simulink model "robobee_smoothSynchAsynch"  (R2021a)
settings: Solver=ode5  StartTime=0.0  StopTime=10  FixedStep=samptime  RelTol=1e-3
values from neighbouring files (symbols this model uses):
  Amplitude = 4    [robobee_simulink_script.m]
  den = [1 a2 a3]    [robobee_simulink_script.m]
  Frequency = 66    [robobee_simulink_script.m]
  num = [a1 0]    [robobee_simulink_script.m]
  pf = [0.0008   -0.0042    0.0029]    [robobee_simulink_script.m]
  samptime = 1/10000    (= 0.0001)    [robobee_simulink_script.m]
  t_end = 6+4    (= 10)    [robobee_simulink_script.m]
  t_switch = t_end/2    (= 5)    [robobee_simulink_script.m]
  VBias = 200/daq_to_piezo_volt    (= 8)    [robobee_simulink_script.m]
undefined symbols (not defined in the file or in its folder): National_Instruments, PCIe
libraries: sldrtlib x3, simulink x2, cstblocks x1
settings Model: SimulationMode=external  ExtModeTrigDuration=500000  Creator=Gravish Lab  LastModifiedBy=RoBeePC
settings SolverCC: AlgebraicLoopSolver=TrustRegion
settings DataIOCC: ReturnWorkspaceOutputs=off
settings DebuggingCC: SFMachineParentedDataDiag=warning  ArithmeticOperatorsInVariantConditions=warning
settings SFSimCC: SimUseLocalCustomCode=off  CustomCodeUndefinedFunction=UseInterfaceOnly
settings RTWCC: Description=Simulink Desktop Real-Time  SystemTargetFile=sldrt.tlc  TemplateMakefile=sldrt.tmf  RTWUseLocalCustomCode=off  RTWCompilerOptimization=on
settings CodeAppCC: MaxIdLength=95  StateflowObjectComments=on
settings SimulinkDesktopRealTimeCC: TargetPreCompLibLocation=C:\Program Files\MATLAB\R2021a\toolbox\sldrt\lib\win64

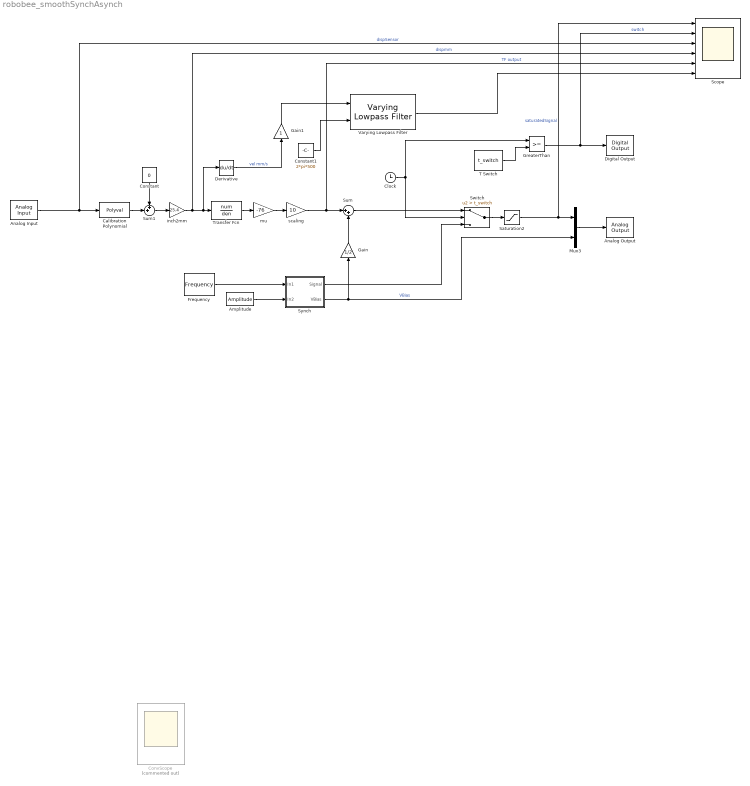
== system robobee_smoothSynchAsynch ==
  Amplitude : Constant  Value=Amplitude
  Analog Input : sldrtlib/Analog Input  SampleTime=samptime  MaxMissedTicks=10  ShowMissedTicks=off  YieldWhenWaiting=off  DrvName=National_Instruments/PCIe-6343  DrvAddress=4294967295  DrvOptions=[0 1 1 0 0 0 0]  Channels=1  RangeMode=1  VoltRange=1  DataType=1
      settings: AttributesFormatString=National Instruments\nPCIe-6343 [auto]
  Analog Output : sldrtlib/Analog Output  SampleTime=samptime  MaxMissedTicks=10  ShowMissedTicks=off  YieldWhenWaiting=off  DrvName=National_Instruments/PCIe-6343  DrvAddress=4294967295  DrvOptions=[0 1 1 0 0 0 0]  Channels=[1,2]  RangeMode=1  VoltRange=1  InitialValue=0  FinalValue=0
      settings: AttributesFormatString=National Instruments\nPCIe-6343 [auto]
  Calibration Polynomial : Polyval  Coefs=pf
  Clock : Clock
  Constant : Constant  Value=0
  Constant1 : Constant  Value=2*pi*500
  ConvScope : Scope  Commented=on  NumInputPorts=5
  Derivative : Derivative
  Digital Output : sldrtlib/Digital Output  SampleTime=samptime  MaxMissedTicks=10  ShowMissedTicks=off  YieldWhenWaiting=off  DrvName=National_Instruments/PCIe-6343  DrvAddress=4294967295  DrvOptions=[0 1 1 0 0 0 0]  Channels=1  BitMode=1  InitialValue=0  FinalValue=0
      settings: AttributesFormatString=National Instruments\nPCIe-6343 [auto]  SourceProductBaseCode=WT
  Frequency : Constant  Value=Frequency
  Gain : Gain  Gain=1/2
  Gain1 : Gain
  GreaterThan : RelationalOperator  OutDataTypeStr=boolean  RndMeth=Simplest
  Mux3 : Mux  Inputs=2
  Saturation2 : Saturate  UpperLimit=8  LowerLimit=0
  Scope : Scope  NumInputPorts=6
  Sum : Sum  Inputs=|++
  Sum1 : Sum  Inputs=++|
  Switch : Switch  Criteria=u2 > Threshold  Threshold=t_switch
  Synch : Subsystem
  T Switch : Constant  Value=t_switch
  Transfer Fcn : TransferFcn  Numerator=num  Denominator=den
  Varying Lowpass Filter : cstblocks/Linear Parameter Varying/Varying Lowpass Filter  N=2
  inch2mm : Gain  Gain=25.4
  mu : Gain  Gain=-76
  scaling : Gain  Gain=10
  wires:
  Saturation2/1 -> Scope/1, Mux3/1  "saturatedSignal"
  Analog Input/1 -> Scope/3, Calibration Polynomial/1  "dispSensor"
  Transfer Fcn/1 -> mu/1
  mu/1 -> scaling/1
  Mux3/1 -> Analog Output/1
  Switch/1 -> Saturation2/1
  Sum/1 -> Switch/1
  Clock/1 -> GreaterThan/1, Switch/2
  inch2mm/1 -> Scope/4, Derivative/1, Transfer Fcn/1  "dispmm"
  Sum1/1 -> inch2mm/1
  T Switch/1 -> GreaterThan/2
  GreaterThan/1 -> Scope/2, Digital Output/1  "switch"
  Frequency/1 -> Synch/1(In1)
  Amplitude/1 -> Synch/2(In2)
  Synch/2(VBias) -> Gain/1, Mux3/2  "VBias"
  Synch/1(Signal) -> Switch/3
  scaling/1 -> Scope/5, Sum/1  "TF output"
  Calibration Polynomial/1 -> Sum1/2
  Constant/1 -> Sum1/1
  Gain/1 -> Sum/2
  Derivative/1 -> Gain1/1  "vel mm/s"
  Gain1/1 -> Varying Lowpass Filter/1
  Constant1/1 -> Varying Lowpass Filter/2
  Varying Lowpass Filter/1 -> Scope/6

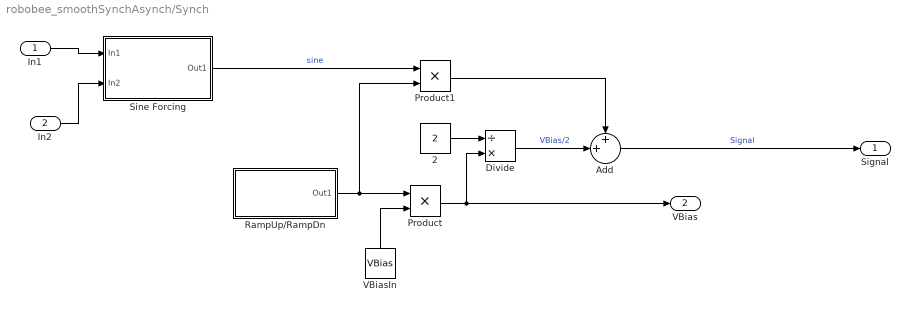
== system robobee_smoothSynchAsynch/Synch ==
  In1 : Inport
  In2 : Inport  Port=2
  "2 " : Constant  Value=2
  Add : Sum  Inputs=++|
  Divide : Product  Inputs=/*
  Product : Product
  Product1 : Product
  RampUp/RampDn : Subsystem
  Sine Forcing : Subsystem
  VBiasIn : Constant  Value=VBias
  Signal : Outport
  VBias : Outport  Port=2
  wires:
  In2/1 -> Sine Forcing/2(In2)
  VBiasIn/1 -> Product/2
  RampUp/RampDn/1(Out1) -> Product/1, Product1/2
  "2 "/1 -> Divide/1
  Product1/1 -> Add/1
  Sine Forcing/1(Out1) -> Product1/1  "sine"
  In1/1 -> Sine Forcing/1(In1)
  Divide/1 -> Add/2  "VBias/2"
  Product/1 -> Divide/2, VBias/1
  Add/1 -> Signal/1  "Signal"

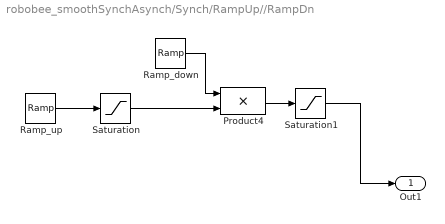
== system robobee_smoothSynchAsynch/Synch/RampUp//RampDn ==
  Product4 : Product
  Ramp_down : simulink/Sources/Ramp  slope=-.5  start=t_end-2  InitialOutput=1
  Ramp_up : simulink/Sources/Ramp  slope=.5  start=0  InitialOutput=0
  Saturation : Saturate  UpperLimit=1  LowerLimit=0
  Saturation1 : Saturate  UpperLimit=1  LowerLimit=0
  Out1 : Outport
  wires:
  Product4/1 -> Saturation1/1
  Ramp_down/1 -> Product4/1
  Saturation/1 -> Product4/2
  Ramp_up/1 -> Saturation/1
  Saturation1/1 -> Out1/1

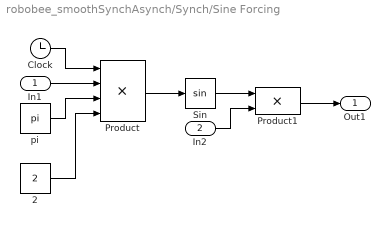
== system robobee_smoothSynchAsynch/Synch/Sine Forcing ==
  In1 : Inport
  In2 : Inport  Port=2
  2 : Constant  Value=2
  Clock : Clock
  Product : Product  Inputs=4
  Product1 : Product
  Sin : Trigonometry  OutputSignalType=real
  pi : Constant  Value=pi
  Out1 : Outport
  wires:
  Sin/1 -> Product1/1
  In2/1 -> Product1/2
  Clock/1 -> Product/1
  Product1/1 -> Out1/1
  2/1 -> Product/4
  pi/1 -> Product/3
  Product/1 -> Sin/1
  In1/1 -> Product/2
